simulink model "compare_linear_vs_non_linear_simulation"  (R2020a)
settings: Solver=ode4  StartTime=0.0  StopTime=80  FixedStep=0.01  RelTol=1e-3
InitFcn:
  | linearize_script;
values from neighbouring files (symbols this model uses):
  Ac = [d_f1_dth,d_f1_dyw,d_f1_dw_th,d_f1_dw_yw ... (first row only)    [linearize_heli.m]    (also in linearize_script.m)
  Bc = [d_f1_Vmp,d_f1_Vmy ... (first row only)    [linearize_heli.m]    (also in linearize_script.m)
  th_op = -10*pi/180    (= -0.174532925199)    [initialize_system.m]    (also in linearize_script.m)
  Vmp_op = (Kyy*m_heli*g*cos(th_op)*l_cm) / (Kyy*Kpp - Kyp*Kpy)    [initialize_system.m]    (also in linearize_script.m)
  Vmy_op = (Kyp*Vmp_op) / (Kyy)    [initialize_system.m]    (also in linearize_script.m)
  w_th_op = 0    [initialize_system.m]    (also in linearize_script.m)
  w_yw_op = 0    [initialize_system.m]    (also in linearize_script.m)
  yw_op = pi/2    (= 1.57079632679)    [initialize_system.m]    (also in linearize_script.m)
libraries: realtime_pacer_lib x1
(part 1 of 2)
settings Model: Creator=engen  LastModifiedBy=eirik.engen

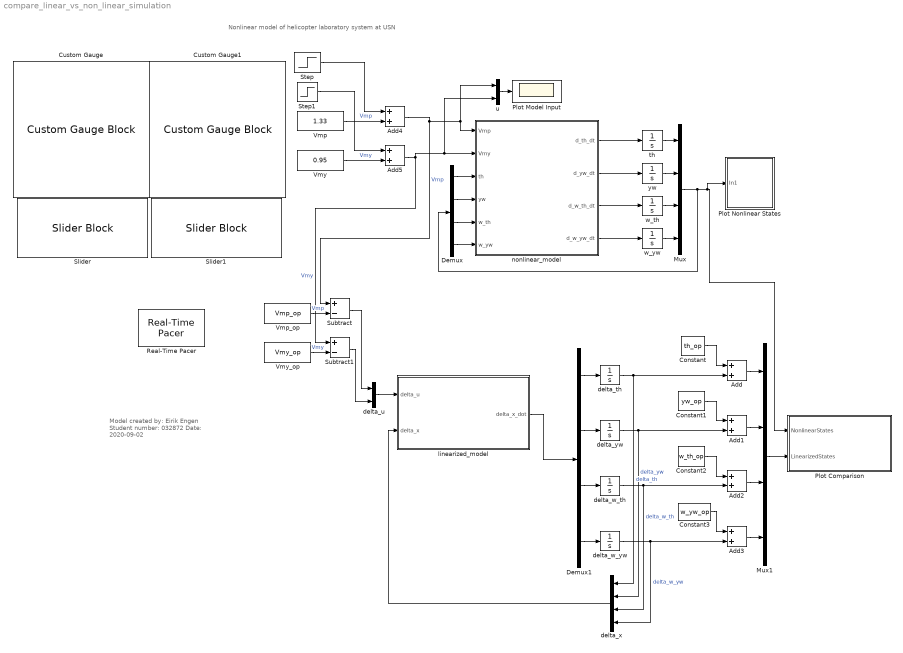
== system compare_linear_vs_non_linear_simulation ==
  note: Model created by: Eirik Engen
      | Student number: 032872
      | Date: 2020-09-02
  note: Nonlinear model of helicopter laboratory system at USN
  Add{,1..5} (6 alike) : Sum
  Constant : Constant  Value=th_op
  Constant1 : Constant  Value=yw_op
  Constant2 : Constant  Value=w_th_op
  Constant3 : Constant  Value=w_yw_op
  Custom Gauge : CustomGaugeBlock  NeedleImage=data:image/svg+xml;base64,PD94bWwgdmVyc2lvbj0iMS4wIiBlbmNvZGluZz0idXRmLTgiPz4KPCEtLSBHZW5lcmF0b3I6IEFkb2JlIElsbHVzdHJhdG9yIDE5LjIuMSwgU1ZHIEV4cG9ydCBQbHVnLUluIC4gU1ZHIFZlcnNpb246IDYuMDAgQnVpbGQgMCkgIC0tPgo8c3ZnIHZlcnNpb249IjEuMSIgeG1sbnM9Imh0dHA6Ly93d3cudzMub3JnLzIwMDAvc3ZnIiB4bWxuczp4bGluaz0iaHR0cDovL3d3dy53My5vcmcvMTk5OS94bGluayIgeD0iMHB4IiB5PSIwcHgiCgkgdmlld0JveD0iMCAwIDIwMCA1MCIgc3R5bGU9ImVuYWJsZS1iYWNrZ3JvdW5kOm5ldyAw ...(+9940 chars)  NeedleXPos=0.3917048004629797  NeedleYPos=0.4829768357659356  NeedleHeight=0.10490569201603188  NeedleWidth=0.1728243811597186  NeedleInitialRotation=-59.94322499147643  BackgroundImage=data:image/svg+xml;base64,PD94bWwgdmVyc2lvbj0iMS4wIiBlbmNvZGluZz0iVVRGLTgiIHN0YW5kYWxvbmU9Im5vIj8+CjwhLS0gR2VuZXJhdG9yOiBBZG9iZSBJbGx1c3RyYXRvciAxOS4yLjEsIFNWRyBFeHBvcnQgUGx1Zy1JbiAuIFNWRyBWZXJzaW9uOiA2LjAwIEJ1aWxkIDApICAtLT4KCjxzdmcKICAgeG1sbnM6ZGM9Imh0dHA6Ly9wdXJsLm9yZy9kYy9lbGVtZW50cy8xLjEvIgogICB4bWxuczpjYz0iaHR0cDovL2NyZWF0aXZlY29tbW9ucy5vcmcvbnMjIgogICB4bWxuczpyZGY9Imh0dHA6Ly93d3cudzMub3JnLzE5OTkvMDIvMjItcmRmLXN5bnRh ...(+9660 chars)  GaugeMax=5  GaugeArcDefined=true  GaugeArcRadius=0.12284021706659634  GaugeArcStrokeWidth=0.03592322137076784  GaugeArcRotation=240.5385250290321  GaugeArcRatio=0.8333333333333  GaugeArcTransparency=0  ValueArcColor=#1759b0  GaugeTickColor=#faf5c8  TickInterval=1  ScaleColorsJSON="[{\"Min\":0,\"Max\":1.1,\"Color\":[1,1,0]},{\"Min\":1.1,\"Max\":1.4,\"Color\":[0,1,0]},{\"Min\":1.4,\"Max\":5,\"Color\":[1,1,0]}]"  fixedAspectRatio=on  IsLinearGauge=false  GaugeTrackLeft=0.35  GaugeTrackTop=0.35  GaugeTrackHeight=0.1  GaugeTrackWidth=0.3  GaugeTrackRotation=0
  Custom Gauge1 : CustomGaugeBlock  NeedleImage=data:image/svg+xml;base64,PD94bWwgdmVyc2lvbj0iMS4wIiBlbmNvZGluZz0idXRmLTgiPz4KPCEtLSBHZW5lcmF0b3I6IEFkb2JlIElsbHVzdHJhdG9yIDE5LjIuMSwgU1ZHIEV4cG9ydCBQbHVnLUluIC4gU1ZHIFZlcnNpb246IDYuMDAgQnVpbGQgMCkgIC0tPgo8c3ZnIHZlcnNpb249IjEuMSIgeG1sbnM9Imh0dHA6Ly93d3cudzMub3JnLzIwMDAvc3ZnIiB4bWxuczp4bGluaz0iaHR0cDovL3d3dy53My5vcmcvMTk5OS94bGluayIgeD0iMHB4IiB5PSIwcHgiCgkgdmlld0JveD0iMCAwIDIwMCA1MCIgc3R5bGU9ImVuYWJsZS1iYWNrZ3JvdW5kOm5ldyAw ...(+9940 chars)  NeedleXPos=0.3917048004629797  NeedleYPos=0.4829768357659356  NeedleHeight=0.10490569201603188  NeedleWidth=0.1728243811597186  NeedleInitialRotation=-59.94322499147643  BackgroundImage=data:image/svg+xml;base64,PD94bWwgdmVyc2lvbj0iMS4wIiBlbmNvZGluZz0iVVRGLTgiIHN0YW5kYWxvbmU9Im5vIj8+CjwhLS0gR2VuZXJhdG9yOiBBZG9iZSBJbGx1c3RyYXRvciAxOS4yLjEsIFNWRyBFeHBvcnQgUGx1Zy1JbiAuIFNWRyBWZXJzaW9uOiA2LjAwIEJ1aWxkIDApICAtLT4KCjxzdmcKICAgeG1sbnM6ZGM9Imh0dHA6Ly9wdXJsLm9yZy9kYy9lbGVtZW50cy8xLjEvIgogICB4bWxuczpjYz0iaHR0cDovL2NyZWF0aXZlY29tbW9ucy5vcmcvbnMjIgogICB4bWxuczpyZGY9Imh0dHA6Ly93d3cudzMub3JnLzE5OTkvMDIvMjItcmRmLXN5bnRh ...(+9660 chars)  GaugeMax=5  GaugeArcDefined=true  GaugeArcRadius=0.12284021706659634  GaugeArcStrokeWidth=0.03592322137076784  GaugeArcRotation=240.5385250290321  GaugeArcRatio=0.8333333333333  GaugeArcTransparency=0  ValueArcColor=#1759b0  GaugeTickColor=#faf5c8  TickInterval=1  ScaleColorsJSON="[{\"Min\":0,\"Max\":0.4,\"Color\":[1,1,0]},{\"Min\":0.4,\"Max\":1.3,\"Color\":[0,1,0]},{\"Min\":1.3,\"Max\":5,\"Color\":[1,1,0]}]"  fixedAspectRatio=on  IsLinearGauge=false  GaugeTrackLeft=0.35  GaugeTrackTop=0.35  GaugeTrackHeight=0.1  GaugeTrackWidth=0.3  GaugeTrackRotation=0
  Demux : Demux
  Demux1 : Demux
  Mux : Mux
  Mux1 : Mux
  Plot Comparison : Subsystem  TreatAsAtomicUnit=on
  Plot Model Input : Scope
  Plot Nonlinear States : Subsystem
  Real-Time Pacer : realtime_pacer_lib/Real-Time Pacer  simTimePerRealTime=10
  Slider : SliderBlock  ScaleMax=1.5
  Slider1 : SliderBlock  ScaleMax=1.5
  Step : Step  Time=20  After=0.02  SampleTime=0
  Step1 : Step  Time=40  After=0.01  SampleTime=0
  Subtract : Sum  Inputs=+-
  Subtract1 : Sum  Inputs=+-
  Vmp : Constant  Value=1.33  SampleTime=-1
  Vmp_op : Constant  Value=Vmp_op  SampleTime=-1
  Vmy : Constant  Value=0.95  SampleTime=-1
  Vmy_op : Constant  Value=Vmy_op  SampleTime=-1
  delta_th : Integrator  ContinuousStateAttributes='w_yw'
  delta_u : Mux  Inputs=2
  delta_w_th : Integrator
  delta_w_yw : Integrator
  delta_x : Mux
  delta_yw : Integrator
  linearized_model : MATLAB Function  TreatAsAtomicUnit=on
  nonlinear_model : MATLAB Function  TreatAsAtomicUnit=on
  th : Integrator  InitialCondition=-10*pi/180  LimitOutput=on  UpperSaturationLimit=45*pi/180  LowerSaturationLimit=-45*pi/180  ContinuousStateAttributes='th'
  u : Mux  Inputs=2
  w_th : Integrator  ContinuousStateAttributes='w_th'
  w_yw : Integrator  ContinuousStateAttributes='w_yw'
  yw : Integrator  InitialCondition=pi/2  LimitOutput=on  UpperSaturationLimit=180*pi/180  LowerSaturationLimit=0  ContinuousStateAttributes='yw'
  wires:
  Add4/1 -> Subtract/1, nonlinear_model/1(Vmp), u/1  "Vmp"
  Add5/1 -> u/2, nonlinear_model/2(Vmy), Subtract1/1  "Vmy"
  nonlinear_model/1(d_th_dt) -> th/1
  nonlinear_model/2(d_yw_dt) -> yw/1
  nonlinear_model/3(d_w_th_dt) -> w_th/1
  nonlinear_model/4(d_w_yw_dt) -> w_yw/1
  th/1 -> Mux/1
  yw/1 -> Mux/2
  w_th/1 -> Mux/3
  w_yw/1 -> Mux/4
  Mux/1 -> Plot Comparison/1(NonlinearStates), Plot Nonlinear States/1(In1), Demux/1
  Demux/1 -> nonlinear_model/3(th)
  Demux/2 -> nonlinear_model/4(yw)
  Demux/3 -> nonlinear_model/5(w_th)
  Demux/4 -> nonlinear_model/6(w_yw)
  u/1 -> Plot Model Input/1
  delta_u/1 -> linearized_model/1(delta_u)
  Vmp_op/1 -> Subtract/2  "Vmp"
  Subtract/1 -> delta_u/1
  Vmy_op/1 -> Subtract1/2  "Vmy"
  Subtract1/1 -> delta_u/2
  linearized_model/1(delta_x_dot) -> Demux1/1
  Demux1/1 -> delta_th/1
  Demux1/2 -> delta_yw/1
  Demux1/3 -> delta_w_th/1
  Demux1/4 -> delta_w_yw/1
  Constant/1 -> Add/1
  Constant1/1 -> Add1/1
  Constant2/1 -> Add2/1
  Constant3/1 -> Add3/1
  Add/1 -> Mux1/1
  Add1/1 -> Mux1/2
  Add2/1 -> Mux1/3
  Add3/1 -> Mux1/4
  Mux1/1 -> Plot Comparison/2(LinearizedStates)
  delta_th/1 -> delta_x/1, Add/2  "delta_th"
  delta_yw/1 -> delta_x/2, Add1/2  "delta_yw"
  delta_w_th/1 -> delta_x/3, Add2/2  "delta_w_th"
  delta_w_yw/1 -> delta_x/4, Add3/2  "delta_w_yw"
  delta_x/1 -> linearized_model/2(delta_x)
  Vmp/1 -> Add4/2  "Vmp"
  Vmy/1 -> Add5/2  "Vmy"
  Step/1 -> Add4/1
  Step1/1 -> Add5/1

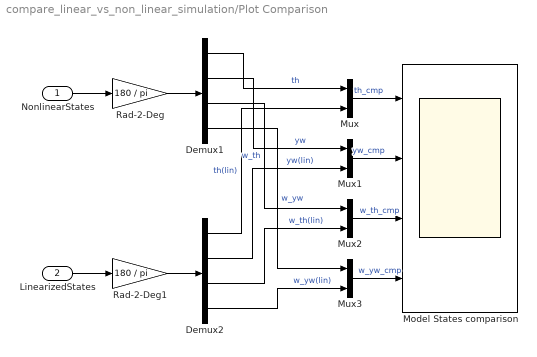
== system compare_linear_vs_non_linear_simulation/Plot Comparison ==
  NonlinearStates : Inport
  LinearizedStates : Inport  Port=2
  Demux1 : Demux
  Demux2 : Demux
  Model States comparison : Scope  NumInputPorts=4
  Mux{,1..3} (4 alike) : Mux  Inputs=2
  Rad-2-Deg : Gain  Gain=180 / pi
  Rad-2-Deg1 : Gain  Gain=180 / pi
  wires:
  NonlinearStates/1 -> Rad-2-Deg/1
  Rad-2-Deg/1 -> Demux1/1
  LinearizedStates/1 -> Rad-2-Deg1/1
  Rad-2-Deg1/1 -> Demux2/1
  Mux/1 -> Model States comparison/1  "th_cmp"
  Mux1/1 -> Model States comparison/2  "yw_cmp"
  Mux2/1 -> Model States comparison/3  "w_th_cmp"
  Mux3/1 -> Model States comparison/4  "w_yw_cmp"
  Demux2/4 -> Mux3/2  "w_yw(lin)"
  Demux1/4 -> Mux3/1  "w_yw"
  Demux2/3 -> Mux2/2  "w_th(lin)"
  Demux1/3 -> Mux2/1  "w_th"
  Demux2/2 -> Mux1/2  "yw(lin)"
  Demux1/2 -> Mux1/1  "yw"
  Demux2/1 -> Mux/2  "th(lin)"
  Demux1/1 -> Mux/1  "th"

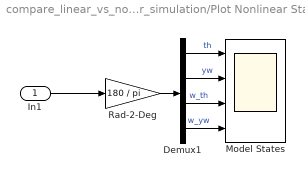
== system compare_linear_vs_non_linear_simulation/Plot Nonlinear States ==
  In1 : Inport
  Demux1 : Demux
  Model States : Scope  NumInputPorts=4
  Rad-2-Deg : Gain  Gain=180 / pi
  wires:
  In1/1 -> Rad-2-Deg/1
  Demux1/2 -> Model States/2  "yw"
  Demux1/3 -> Model States/3  "w_th"
  Demux1/1 -> Model States/1  "th"
  Demux1/4 -> Model States/4  "w_yw"
  Rad-2-Deg/1 -> Demux1/1

== matlab function compare_linear_vs_non_linear_simulation/linearized_model ==
  data: delta_u input; delta_x_dot output; delta_x input; Ac parameter; Bc parameter
% Simulink linearized model of USN helicopter
% Author: Eirik Engen
% Date: 2020-09-02

function delta_x_dot  = linearized_model(delta_u, delta_x, Ac, Bc)

delta_x_dot = Ac*delta_x + Bc*delta_u;
